simulink model "sysp7_LC"  (R2023a)
settings: Solver=ode15s  StartTime=0.0  StopTime=30  MaxStep=1E-3  RelTol=1E-3
libraries: slpidlib x1
settings Model: Creator=Ariel  LastModifiedBy=Ariel
settings DataIOCC: ReturnWorkspaceOutputs=off  TimeSaveName=t
settings DebuggingCC: AlgebraicLoopMsg=none  ArtificialAlgebraicLoopMsg=none  MaxConsecutiveZCsMsg=none  ModelReferenceExtraNoncontSigs=none  OperatingPointInterfaceChecksumMismatchMsg=none

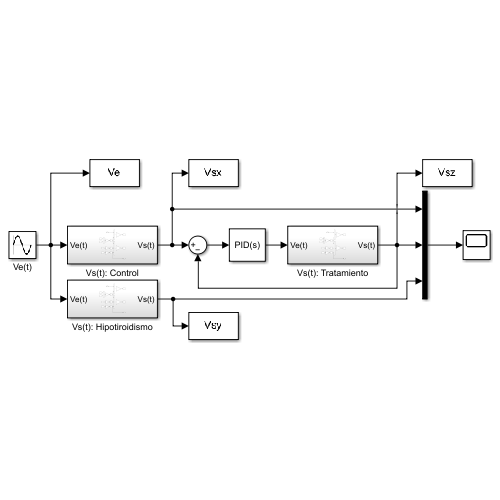
[thumbnail: Simulink's stored preview of the top-level diagram]
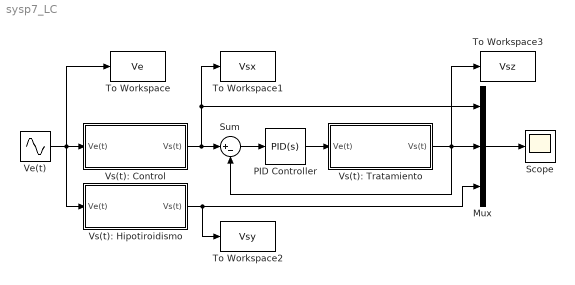
== system sysp7_LC ==
  Mux : Mux  Inputs=3
  PID Controller : slpidlib/PID Controller  Controller=PID  Form=Parallel  TimeDomain=Continuous-time  UseExternalTs=off  SampleTime=-1  IntegratorMethod=Forward Euler  FilterMethod=Forward Euler  ControllerParametersSource=internal  P=1508.7022  I=12301.4891  UseKiTs=off  D=44.8051  N=10  UseFilter=on  TunerSelectOption=Transfer Function Based (PID Tuner App)  InitialConditionSource=internal  InitialConditionForIntegrator=0  InitialConditionForFilter=0  DifferentiatorICPrevScaledInput=0  ExternalReset=none  TrackingMode=off  Kt=1  LimitOutput=off  SatLimitsSource=internal  UpperSaturationLimit=inf  LowerSaturationLimit=-inf  LinearizeAsGain=on  AntiWindupMode=none  Kb=1  LimitIntegrator=off  UpperIntegratorSaturationLimit=inf  LowerIntegratorSaturationLimit=-inf  POutMin=[]  POutMax=[]  IOutMin=[]  IOutMax=[]  DOutMin=[]  DOutMax=[]  NOutMin=[]  NOutMax=[]  SumOutMin=[]  SumOutMax=[]  SaturationOutMin=[]  SaturationOutMax=[]  PParamMin=[]  PParamMax=[]  IParamMin=[]  IParamMax=[]  DParamMin=[]  DParamMax=[]  NParamMin=[]  NParamMax=[]  KbParamMin=[]  KbParamMax=[]  KtParamMin=[]  KtParamMax=[]  KbOutMin=[]  KbOutMax=[]  KtOutMin=[]  KtOutMax=[]  IntegratorOutMin=[]  IntegratorOutMax=[]  FilterOutMin=[]  FilterOutMax=[]  SumI1OutMin=[]  SumI1OutMax=[]  SumI2OutMin=[]  SumI2OutMax=[]  SumI3OutMin=[]  SumI3OutMax=[]  SumI4OutMin=[]  SumI4OutMax=[]  SumDOutMin=[]  SumDOutMax=[]  DifferentiatorOutMin=[]  DifferentiatorOutMax=[]  FilterDiffOutCoefMin=[]  FilterDiffOutCoefMax=[]  ReciprocalOutMin=[]  ReciprocalOutMax=[]  SumDenOutMin=[]  SumDenOutMax=[]  SumNumOutMin=[]  SumNumOutMax=[]  DivideOutMin=[]  DivideOutMax=[]  UdiffTsProdOutMin=[]  UdiffTsProdOutMax=[]  NTsProdOutMin=[]  NTsProdOutMax=[]  UintegralTsProdOutMin=[]  UintegralTsProdOutMax=[]  UngainTsProdOutMin=[]  UngainTsProdOutMax=[]  ClampingZeroOutDataTypeStr=Inherit: Inherit via back propagation  ClampingZeroOutMin=[]  ClampingZeroOutMax=[]  FilterDenConstantOutDataTypeStr=Inherit: Inherit via back propagation  FilterDenConstantOutMin=[]  FilterDenConstantOutMax=[]  PCopyOutDataTypeStr=Inherit: Inherit via back propagation  PCopyOutMin=[]  PCopyOutMax=[]  NCopyOutDataTypeStr=Inherit: Inherit via back propagation  NCopyOutMin=[]  NCopyOutMax=[]  IntegratorContinuousStateAttributes=''  IntegratorStateMustResolveToSignalObject=off  IntegratorRTWStateStorageClass=Auto  FilterContinuousStateAttributes=''  FilterStateMustResolveToSignalObject=off  FilterRTWStateStorageClass=Auto  ParallelPVariant=InternalParameters  IdealPVariant=Disabled  IVariant=InternalParameters  DVariant=InternalParameters  IntegratorVariant=Continuous  SatVariant=Disabled  AWVariant=Passthrough  PCopyVariant=Disabled  TRVariant=Disabled  FdbkBlocksVariant=Forward  IdealPFdbkVariant=Disabled  SatFdbkVariant=Disabled  DerivativeFilterVariant=ContFilter  NVariant=InternalParameters  NCopyVariant=Disabled  FilterICVariant=InternalICsFilter  IntegratorICVariant=InternalICs  ExternalResetVariant=Disabled  TRSumVariant=Passthrough  SumFdbkVariant=Disabled  SumVariant=Sum_PID  TsampFilterVariant=InternalTs  TsampNgainVariant=Passthrough  TsampIntegralVariant=Disabled_SignalSpec  ExternalSaturationOutDataTypeStr=Inherit: Same as second input
  Scope : Scope
  Sum : Sum  Inputs=|+-
  To Workspace : ToWorkspace  VariableName=Ve  SaveFormat=Timeseries  SampleTime=-1
  To Workspace1 : ToWorkspace  VariableName=Vsx  SaveFormat=Timeseries  SampleTime=-1
  To Workspace2 : ToWorkspace  VariableName=Vsy  SaveFormat=Timeseries  SampleTime=-1
  To Workspace3 : ToWorkspace  VariableName=Vsz  SaveFormat=Timeseries  SampleTime=-1
  Ve(t) : Sin  Frequency=pi/2  SampleTime=0
  Vs(t): Control : Subsystem
  Vs(t): Hipotiroidismo : Subsystem
  Vs(t): Tratamiento : Subsystem
  wires:
  Mux/1 -> Scope/1
  Vs(t): Control/1(Vs(t)) -> Mux/1, To Workspace1/1, Sum/1
  Sum/1 -> PID Controller/1
  PID Controller/1 -> Vs(t): Tratamiento/1(Ve(t))
  Vs(t): Tratamiento/1(Vs(t)) -> To Workspace3/1, Mux/2, Sum/2
  Vs(t): Hipotiroidismo/1(Vs(t)) -> To Workspace2/1, Mux/3
  Ve(t)/1 -> Vs(t): Hipotiroidismo/1(Ve(t)), Vs(t): Control/1(Ve(t)), To Workspace/1

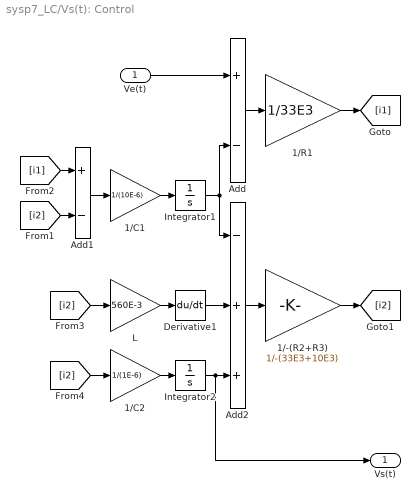
== system sysp7_LC/Vs(t): Control ==
  Ve(t) : Inport
  1/-(R2+R3) : Gain  Gain=1/-(33E3+10E3)
  1/C1 : Gain  Gain=1/(10E-6)
  1/C2 : Gain  Gain=1/(1E-6)
  1/R1 : Gain  Gain=1/33E3
  Add : Sum  Inputs=+-
  Add1 : Sum  Inputs=+-
  Add2 : Sum  Inputs=-++
  Derivative1 : Derivative
  Integrator1 : Integrator
  Integrator2 : Integrator
  L : Gain  Gain=560E-3
  Vs(t) : Outport
  wires:
  Ve(t)/1 -> Add/1
  Add1/1 -> 1/C1/1
  [i1] -> Add1/1
  [i2] -> Add1/2
  Add/1 -> 1/R1/1
  1/R1/1 -> [i1]
  Integrator1/1 -> Add/2, Add2/1
  1/C1/1 -> Integrator1/1
  [i2] -> L/1
  L/1 -> Derivative1/1
  1/C2/1 -> Integrator2/1
  [i2] -> 1/C2/1
  Integrator2/1 -> Vs(t)/1, Add2/3
  Derivative1/1 -> Add2/2
  Add2/1 -> 1/-(R2+R3)/1
  1/-(R2+R3)/1 -> [i2]

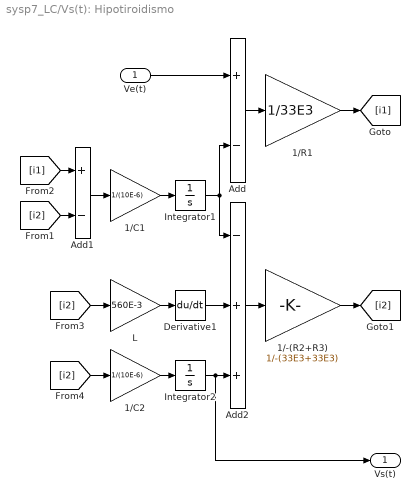
== system sysp7_LC/Vs(t): Hipotiroidismo ==
  Ve(t) : Inport
  1/-(R2+R3) : Gain  Gain=1/-(33E3+33E3)
  1/C1 : Gain  Gain=1/(10E-6)
  1/C2 : Gain  Gain=1/(10E-6)
  1/R1 : Gain  Gain=1/33E3
  Add : Sum  Inputs=+-
  Add1 : Sum  Inputs=+-
  Add2 : Sum  Inputs=-++
  Derivative1 : Derivative
  Integrator1 : Integrator
  Integrator2 : Integrator
  L : Gain  Gain=560E-3
  Vs(t) : Outport
  wires:
  Ve(t)/1 -> Add/1
  Add1/1 -> 1/C1/1
  [i1] -> Add1/1
  [i2] -> Add1/2
  Add/1 -> 1/R1/1
  1/R1/1 -> [i1]
  Integrator1/1 -> Add/2, Add2/1
  1/C1/1 -> Integrator1/1
  [i2] -> L/1
  L/1 -> Derivative1/1
  1/C2/1 -> Integrator2/1
  [i2] -> 1/C2/1
  Integrator2/1 -> Vs(t)/1, Add2/3
  Derivative1/1 -> Add2/2
  Add2/1 -> 1/-(R2+R3)/1
  1/-(R2+R3)/1 -> [i2]

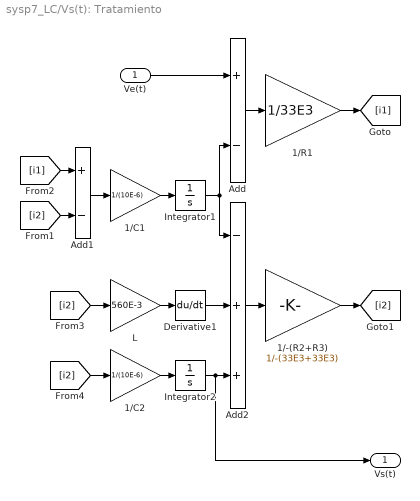
== system sysp7_LC/Vs(t): Tratamiento ==
  Ve(t) : Inport
  1/-(R2+R3) : Gain  Gain=1/-(33E3+33E3)
  1/C1 : Gain  Gain=1/(10E-6)
  1/C2 : Gain  Gain=1/(10E-6)
  1/R1 : Gain  Gain=1/33E3
  Add : Sum  Inputs=+-
  Add1 : Sum  Inputs=+-
  Add2 : Sum  Inputs=-++
  Derivative1 : Derivative
  Integrator1 : Integrator
  Integrator2 : Integrator
  L : Gain  Gain=560E-3
  Vs(t) : Outport
  wires:
  Ve(t)/1 -> Add/1
  Add1/1 -> 1/C1/1
  [i1] -> Add1/1
  [i2] -> Add1/2
  Add/1 -> 1/R1/1
  1/R1/1 -> [i1]
  Integrator1/1 -> Add/2, Add2/1
  1/C1/1 -> Integrator1/1
  [i2] -> L/1
  L/1 -> Derivative1/1
  1/C2/1 -> Integrator2/1
  [i2] -> 1/C2/1
  Integrator2/1 -> Vs(t)/1, Add2/3
  Derivative1/1 -> Add2/2
  Add2/1 -> 1/-(R2+R3)/1
  1/-(R2+R3)/1 -> [i2]
